simulink library "target_gen_lib_seattle"  (R2018b)
settings: Solver=VariableStepAuto  StartTime=0.0  StopTime=10.0  RelTol=1e-3
undefined symbols (not defined in the file): fswParams
libraries: sharedtransform x1, vrlib x1
settings Model: Creator=colem  LastModifiedBy=colem

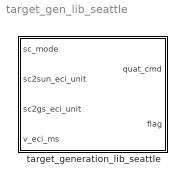
== system target_gen_lib_seattle ==
  target_generation_lib_seattle : Subsystem

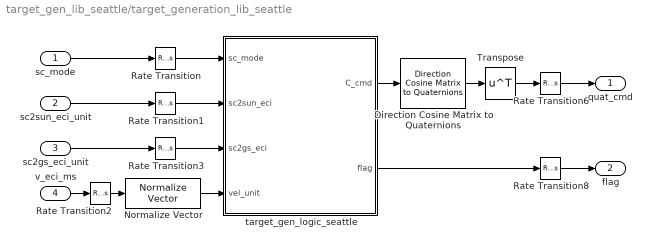
== system target_gen_lib_seattle/target_generation_lib_seattle ==
  sc_mode : Inport
  sc2sun_eci_unit : Inport  Port=2
  sc2gs_eci_unit : Inport  Port=3
  v_eci_ms : Inport  Port=4
  Direction Cosine Matrix to Quaternions : sharedtransform/Direction Cosine Matrix  to Quaternions  aMode=0  action=None  tolerance=eps(2)
      settings: SourceProductName=Aerospace Blockset  SourceProductBaseCode=AE
  Normalize Vector : vrlib/Utilities/Normalize Vector  maxzero=0
      settings: SourceProductName=Simulink 3D Animation  SourceProductBaseCode=VR
  Rate Transition : RateTransition  InitialCondition=fswParams.mode_select.sc_mode_ic  OutPortSampleTime=fswParams.sample_time_s
  Rate Transition1 : RateTransition  OutPortSampleTime=fswParams.sample_time_s
  Rate Transition2 : RateTransition  OutPortSampleTime=fswParams.sample_time_s
  Rate Transition3 : RateTransition  OutPortSampleTime=fswParams.sample_time_s
  Rate Transition6 : RateTransition  InitialCondition=fswParams.controllers.reorientation.qd
  Rate Transition8 : RateTransition
  Transpose : Math  Operator=transpose  SaturateOnIntegerOverflow=on
  target_gen_logic_seattle : MATLAB Function  TreatAsAtomicUnit=on
  quat_cmd : Outport
  flag : Outport  Port=2
  wires:
  Rate Transition8/1 -> flag/1
  sc2gs_eci_unit/1 -> Rate Transition3/1
  Rate Transition1/1 -> target_gen_logic_seattle/2(sc2sun_eci)
  target_gen_logic_seattle/2(flag) -> Rate Transition8/1
  Rate Transition3/1 -> target_gen_logic_seattle/3(sc2gs_eci)
  sc_mode/1 -> Rate Transition/1
  sc2sun_eci_unit/1 -> Rate Transition1/1
  Rate Transition/1 -> target_gen_logic_seattle/1(sc_mode)
  v_eci_ms/1 -> Rate Transition2/1
  Rate Transition2/1 -> Normalize Vector/1
  Normalize Vector/1 -> target_gen_logic_seattle/4(vel_unit)
  target_gen_logic_seattle/1(C_cmd) -> Direction Cosine Matrix to Quaternions/1
  Direction Cosine Matrix to Quaternions/1 -> Transpose/1
  Transpose/1 -> Rate Transition6/1
  Rate Transition6/1 -> quat_cmd/1

== matlab function target_gen_lib_seattle/target_generation_lib_seattle/target_gen_logic_seattle ==
  data: sc_mode input size=1; C_cmd output size=[3 3]; sc2sun_eci input size=3; sc2gs_eci input size=3; flag output; vel_unit input
function [C_cmd,flag]   = target_gen(sc_mode,sc2sun_eci,sc2gs_eci, vel_unit)
% FSW Target Generation Library
%
% Computes desired quaternion depending on the sc_mode
%   mode_logic.low_power        = 1; "safe mode"
%   mode_logic.idle             = 2; "idle/standby mode"
%   mode_logic.stabilize        = 3;
%   mode_logic.nominal          = 4;
%       nominal.desat           = 41;
%       nominal.sun_seek        = 42;
%   mode_logic.point            = 5;
%       point.com               = 51;
%       point.image             = 52;
%       point.exp               = 53;
%
%   Author: Cole Morgan 9/09/2019

% Constants
COM     = [ 0.0; 0.0; 1.0 ]; % COMM antenna boresight vector (F_body)
IMG     = [ 0.0; 0.0; -1.0]; % image camera boresight vector (F_body)
SP      = [ 0.0; 1.0; 0.0 ]; % solar panel boresight vector (F_body)
flag    = 0;
tol     = 1e-3;
Cx5     = [ 1 0 0; 0 cosd(5) sind(5); 0 -sind(5) cosd(5)]; % 5-deg roll
C_cmd   = eye(3);            % initialize target attitude

% Uncomment for testing only %   
% SP      = [1;3;0];
% -------------------------- %

% Validity Checks
if(norm(sc2sun_eci) < tol || norm(sc2gs_eci) < tol )
    sc2sun_unit     = zeros(3,1);
    sc2gs_unit      = zeros(3,1);
    flag = -1;
else
    % Compute unit vectors
    sc2sun_unit = sc2sun_eci./norm(sc2sun_eci);
    sc2gs_unit  = sc2gs_eci./norm(sc2gs_eci);
    % Check for parallel unit vectors
    if ( abs(dot(vel_unit,sc2gs_unit)) > 1-tol ...
                            || abs(dot(sc2sun_unit,sc2gs_unit)) > 1-tol )
        flag = -1;
    end
end

% Main Code
if( sc_mode == 52 && flag == 0 )
    
    % Body vectors
    B1      = IMG;
    B2      = SP;
    Xtb     = B1;
    Ytb     = cross(B1,B2)/norm(cross(B1,B2));
    Ztb     = cross(B1,Ytb)/norm(cross(B1,Ytb));
    
    % Inertial vectors
    S1      = sc2gs_unit;
    S2      = sc2sun_unit;
    Xti     = S1;
    Yti     = cross(S1,S2)/norm(cross(S1,S2));
    Zti     = cross(S1,Yti)/norm(cross(S1,Yti));
    
    % Stack vectors
    Cb  = [Xtb, Ytb, Ztb];
    Ci  = [Xti, Yti, Zti];
    
    % Commanded DCM ( body to inertial )
    C_cmd   = Cb*Ci';
        
elseif( (sc_mode == 42 || sc_mode == 51)  && flag == 0 )
    
    % Tilted so doesn't aling with COM2 -- chose a 5[deg] roll.
%     SP      = Cx5*[0;1;0]; 
    
    % Body
    B1      = COM;
    B2      = SP./norm(SP);
    Xtb     = B1;
    Ytb     = cross(B1,B2)/norm(cross(B1,B2));
    Ztb     = cross(B1,Ytb)/norm(cross(B1,Ytb));
    
    % Inertial
    S1      = sc2gs_unit;
    S2      = sc2sun_unit;
    Xti     = S1;
    Yti     = cross(S1,S2)/norm(cross(S1,S2));
    Zti     = cross(S1,Yti)/norm(cross(S1,Yti));
    
    % Stack vectors
    Cb  = [Xtb, Ytb, Ztb];
    Ci  = [Xti, Yti, Zti];
    
    % Commanded DCM ( body to inertial )
    C_cmd   = Cb*Ci';
 
else
    
    C_cmd   = eye(3);
    
end

% Compute commanded quaternion from DCM
% q_cmd   = dcm2quat( C_cmd );


end
